simulink model "motorFromScratch"  (R2013b)
settings: Solver=ode45  StartTime=0.0  StopTime=10.0  RelTol=1e-3
values from neighbouring files (symbols this model uses):
  Ba = 0.000743    [bradMotor.m]
  Bl = .0037    (= 0.0037)    [commercialMotor.m]
  Jma = 8.1837e-05    [bradMotor.m]
  Jml = .000072    (= 7.2e-05)    [commercialMotor.m]
  Kda = 0.029    [bradMotor.m]
  Kdl = 0.0463    [commercialMotor.m]
  Kea = 0.0240    (= 0.024)    [bradMotor.m]
  Kel = 0.05    [commercialMotor.m]
  La = 14/1000    (= 0.014)    [bradMotor.m]
  Ll = 6/1000    (= 0.006)    [commercialMotor.m]
  Ra = 21.9    [bradMotor.m]
  Rl = 6.6    [commercialMotor.m]
libraries: simulink x2
settings Model: Creator=Maxim  LastModifiedBy=Maxim

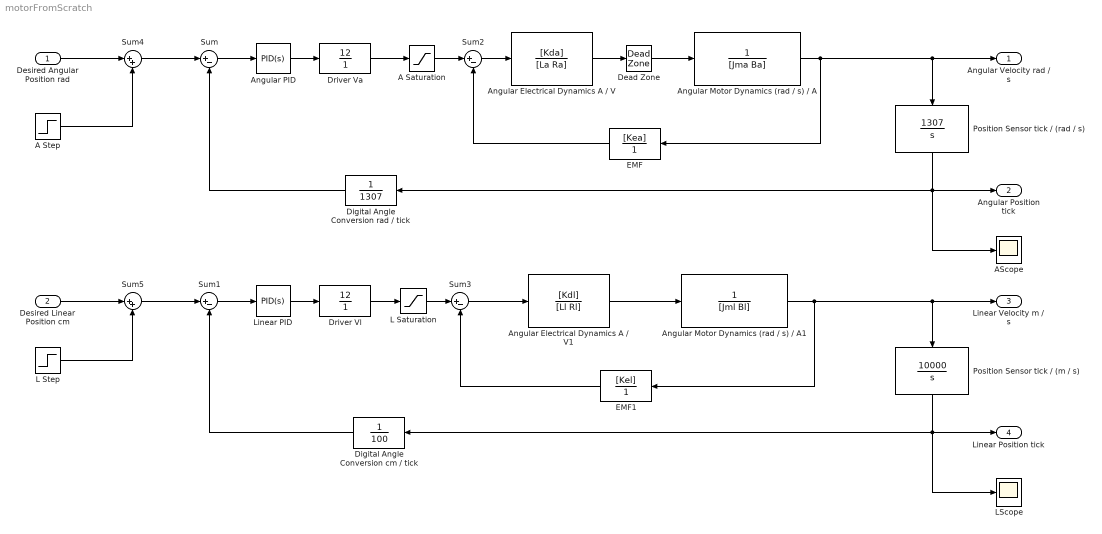
== system motorFromScratch ==
  Desired Angular Position rad : Inport
  Desired Linear Position cm : Inport  Port=2
  A Saturation : Saturate  UpperLimit=6  LowerLimit=-6
  A Step : Step  SampleTime=0
  AScope : Scope
  Angular Electrical Dynamics A / V : TransferFcn  Numerator=[Kda]  Denominator=[La Ra]
  Angular Electrical Dynamics A / V1 : TransferFcn  Numerator=[Kdl]  Denominator=[Ll Rl]
  Angular Motor Dynamics (rad / s) / A : TransferFcn  Denominator=[Jma Ba]
  Angular Motor Dynamics (rad / s) / A1 : TransferFcn  Denominator=[Jml Bl]
  Angular PID : simulink/Continuous/PID Controller  Controller=PID  TimeDomain=Continuous-time  SampleTime=1  IntegratorMethod=Forward Euler  FilterMethod=Forward Euler  Form=Parallel  P=5  I=0  D=1  N=100  InitialConditionSource=internal  InitialConditionForIntegrator=0  InitialConditionForFilter=0  ExternalReset=none  LimitOutput=off  UpperSaturationLimit=inf  LowerSaturationLimit=-inf  LinearizeAsGain=off  AntiWindupMode=none  Kb=1  TrackingMode=off  Kt=1  PParamMin=[]  PParamMax=[]  IParamMin=[]  IParamMax=[]  DParamMin=[]  DParamMax=[]  NParamMin=[]  NParamMax=[]  KbParamMin=[]  KbParamMax=[]  KtParamMin=[]  KtParamMax=[]  POutMin=[]  POutMax=[]  IOutMin=[]  IOutMax=[]  DOutMin=[]  DOutMax=[]  NOutMin=[]  NOutMax=[]  KbOutMin=[]  KbOutMax=[]  KtOutMin=[]  KtOutMax=[]  IntegratorOutMin=[]  IntegratorOutMax=[]  FilterOutMin=[]  FilterOutMax=[]  SumOutMin=[]  SumOutMax=[]  SumI1OutMin=[]  SumI1OutMax=[]  SumI2OutMin=[]  SumI2OutMax=[]  SumI3OutMin=[]  SumI3OutMax=[]  SumDOutMin=[]  SumDOutMax=[]  SaturationOutMin=[]  SaturationOutMax=[]  IntegratorContinuousStateAttributes=''  IntegratorStateMustResolveToSignalObject=off  IntegratorRTWStateStorageClass=Auto  FilterContinuousStateAttributes=''  FilterStateMustResolveToSignalObject=off  FilterRTWStateStorageClass=Auto
  Dead Zone : DeadZone  LowerValue=-0.13  UpperValue=0.13  SaturateOnIntegerOverflow=on
  Digital Angle Conversion cm / tick : TransferFcn  Denominator=[100]
  Digital Angle Conversion rad / tick : TransferFcn  Denominator=[1307]
  Driver Va : TransferFcn  Numerator=[12]  Denominator=[1]
  Driver Vl : TransferFcn  Numerator=[12]  Denominator=[1]
  EMF : TransferFcn  Numerator=[Kea]  Denominator=[1]
  EMF1 : TransferFcn  Numerator=[Kel]  Denominator=[1]
  L Saturation : Saturate  UpperLimit=12  LowerLimit=-12
  L Step : Step  SampleTime=0
  "LScope " : Scope
  Linear PID : simulink/Continuous/PID Controller  Controller=PID  TimeDomain=Continuous-time  SampleTime=1  IntegratorMethod=Forward Euler  FilterMethod=Forward Euler  Form=Parallel  P=5  I=0.03  D=1  N=100  InitialConditionSource=internal  InitialConditionForIntegrator=0  InitialConditionForFilter=0  ExternalReset=none  LimitOutput=off  UpperSaturationLimit=inf  LowerSaturationLimit=-inf  LinearizeAsGain=off  AntiWindupMode=none  Kb=1  TrackingMode=off  Kt=1  PParamMin=[]  PParamMax=[]  IParamMin=[]  IParamMax=[]  DParamMin=[]  DParamMax=[]  NParamMin=[]  NParamMax=[]  KbParamMin=[]  KbParamMax=[]  KtParamMin=[]  KtParamMax=[]  POutMin=[]  POutMax=[]  IOutMin=[]  IOutMax=[]  DOutMin=[]  DOutMax=[]  NOutMin=[]  NOutMax=[]  KbOutMin=[]  KbOutMax=[]  KtOutMin=[]  KtOutMax=[]  IntegratorOutMin=[]  IntegratorOutMax=[]  FilterOutMin=[]  FilterOutMax=[]  SumOutMin=[]  SumOutMax=[]  SumI1OutMin=[]  SumI1OutMax=[]  SumI2OutMin=[]  SumI2OutMax=[]  SumI3OutMin=[]  SumI3OutMax=[]  SumDOutMin=[]  SumDOutMax=[]  SaturationOutMin=[]  SaturationOutMax=[]  IntegratorContinuousStateAttributes=''  IntegratorStateMustResolveToSignalObject=off  IntegratorRTWStateStorageClass=Auto  FilterContinuousStateAttributes=''  FilterStateMustResolveToSignalObject=off  FilterRTWStateStorageClass=Auto
  Position Sensor tick / (m / s) : TransferFcn  Numerator=[10000]  Denominator=[1 0]
  Position Sensor tick / (rad / s) : TransferFcn  Numerator=[1307]  Denominator=[1 0]
  Sum{,1..3} (4 alike) : Sum  Inputs=|+-
  Sum4 : Sum  Inputs=|++
  Sum5 : Sum  Inputs=|++
  "Angular Velocity rad / s " : Outport
  Angular Position tick : Outport  Port=2
  Linear Velocity m / s : Outport  Port=3
  Linear Position tick : Outport  Port=4
  wires:
  Angular PID/1 -> Driver Va/1
  Sum/1 -> Angular PID/1
  Position Sensor tick / (rad / s)/1 -> AScope/1, Digital Angle Conversion rad / tick/1, Angular Position tick/1
  Digital Angle Conversion rad / tick/1 -> Sum/2
  Linear PID/1 -> Driver Vl/1
  Sum1/1 -> Linear PID/1
  Position Sensor tick / (m / s)/1 -> "LScope "/1, Digital Angle Conversion cm / tick/1, Linear Position tick/1
  Digital Angle Conversion cm / tick/1 -> Sum1/2
  EMF/1 -> Sum2/2
  Sum2/1 -> Angular Electrical Dynamics A / V/1
  A Saturation/1 -> Sum2/1
  Driver Va/1 -> A Saturation/1
  Dead Zone/1 -> Angular Motor Dynamics (rad / s) / A/1
  Angular Electrical Dynamics A / V/1 -> Dead Zone/1
  EMF1/1 -> Sum3/2
  Sum3/1 -> Angular Electrical Dynamics A / V1/1
  Angular Electrical Dynamics A / V1/1 -> Angular Motor Dynamics (rad / s) / A1/1
  Angular Motor Dynamics (rad / s) / A1/1 -> Position Sensor tick / (m / s)/1, Linear Velocity m / s/1, EMF1/1
  Angular Motor Dynamics (rad / s) / A/1 -> Position Sensor tick / (rad / s)/1, "Angular Velocity rad / s "/1, EMF/1
  L Saturation/1 -> Sum3/1
  Driver Vl/1 -> L Saturation/1
  Desired Angular Position rad/1 -> Sum4/1
  Sum4/1 -> Sum/1
  A Step/1 -> Sum4/2
  L Step/1 -> Sum5/2
  Sum5/1 -> Sum1/1
  Desired Linear Position cm/1 -> Sum5/1
